simulink model "signal_chooser"  (R2019a)
settings: Solver=VariableStepAuto  StartTime=0.0  StopTime=10.0  RelTol=1e-3
libraries: dspsrcs4 x1, simulink x1
settings Model: Creator=tyson  LastModifiedBy=tyson

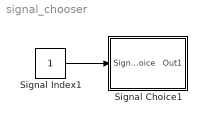
== system signal_chooser ==
  Signal Choice1 : Subsystem  Description=Input Signal
  Signal Index1 : Constant
  wires:
  Signal Index1/1 -> Signal Choice1/1(Signal Choice)

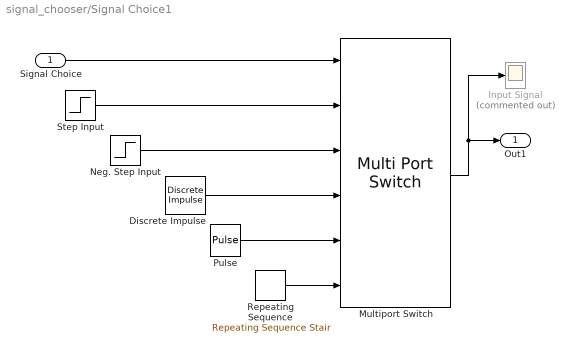
== system signal_chooser/Signal Choice1 ==
  Signal Choice : Inport
  Discrete Impulse : dspsrcs4/Discrete  Impulse  Delay=0  SampleTime=1  FrameSample=1  OutputFrames=off  dataType=double  isSigned=on  wordLen=16  udDataType=sfix(16)  fracBitsMode=Best precision  numFracBits=15  OutDataTypeStr=double  LastOutDataTypeStr=double
  Input Signal : Scope  Commented=on
  Multiport Switch : MultiPortSwitch  Inputs=5
  Neg. Step Input : Step  Time=0  After=-1  SampleTime=0
  "Pulse " : DiscretePulseGenerator  PulseType=Time based  Period=40  PulseWidth=50
  "Repeating Sequence " : simulink/Sources/Repeating Sequence Stair  OutValues=[1 1 1 1 1 0 0 0 0 0 -1 -1 -1 -1 -1 0 0 0 0 0].'  tsamp=-1  OutMin=[]  OutMax=[]  OutDataTypeStr=double  OutputDataTypeScalingMode=double  OutDataType=fixdt(0,8)  ConRadixGroup=Best Precision: Vector-wise  OutScaling=2^-12
  Step Input : Step  Time=0  SampleTime=0
  Out1 : Outport
  wires:
  Step Input/1 -> Multiport Switch/2
  Signal Choice/1 -> Multiport Switch/1
  Multiport Switch/1 -> Input Signal/1, Out1/1
  Neg. Step Input/1 -> Multiport Switch/3
  Discrete Impulse/1 -> Multiport Switch/4
  "Pulse "/1 -> Multiport Switch/5
  "Repeating Sequence "/1 -> Multiport Switch/6
